simulink model "rotation_c"  (R2020a)
settings: Solver=VariableStepAuto  StartTime=0.0  StopTime=10.0  RelTol=1e-3
values from neighbouring files (symbols this model uses):
  euler_angles_NfromB_0_deg = [0; 0; 0]    [p1partApartI.m]
  omega_BwrtN_rps = deg2rad([0; 0; 0.01])    [p1partApartI.m]
libraries: coordinate_transforms x3
settings Model: Creator=Nikita  LastModifiedBy=Nikita

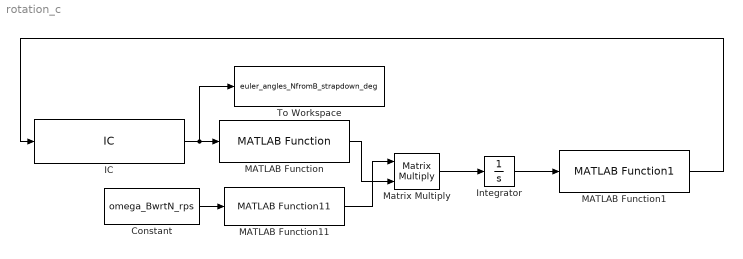
== system rotation_c ==
  Constant : Constant  Value=omega_BwrtN_rps
  IC : InitialCondition  Value=euler_angles_NfromB_0_deg
  Integrator : Integrator
  MATLAB Function : coordinate_transforms/MATLAB Function  SystemSampleTime=-1  Latency=0  AutoFrameSizeCalculation=off
  MATLAB Function1 : coordinate_transforms/MATLAB Function1  SystemSampleTime=-1  Latency=0  AutoFrameSizeCalculation=off
  MATLAB Function11 : coordinate_transforms/MATLAB Function11  SystemSampleTime=-1  Latency=0  AutoFrameSizeCalculation=off
      settings: SourceProductBaseCode=SL
  Matrix Multiply : Product  Multiplication=Matrix(*)
  To Workspace : ToWorkspace  VariableName=euler_angles_NfromB_strapdown_deg  SampleTime=-1
  wires:
  IC/1 -> To Workspace/1, MATLAB Function/1
  Constant/1 -> MATLAB Function11/1
  Matrix Multiply/1 -> Integrator/1
  Integrator/1 -> MATLAB Function1/1
  MATLAB Function1/1 -> IC/1
  MATLAB Function/1 -> Matrix Multiply/2
  MATLAB Function11/1 -> Matrix Multiply/1
